simulink model "TRN_current"  (Simulink 6.2)
settings: Solver=ode45  SolverMode=SingleTasking  StartTime=0  StopTime=6  MaxStep=0.1  RelTol=1e-3  AbsTol=1e-3
libraries: simulink x1
(part 3 of 3)

== system TRN_current/Basal Ganglia/STN/STN discrete model/2 input channel1/leaky integration ==
  Inport : Inport  Port=1  LatchInput=off
  Gain : Gain  Gain=A_rate  SaturateOnIntegerOverflow=on
  Integrator : Integrator
  decay const : Gain  Orientation=left  Gain=-A_rate  SaturateOnIntegerOverflow=on
  sum : Sum  SaturateOnIntegerOverflow=on  InputSameDT=on
  Outport : Outport  InitialOutput=0
  wires:
  Gain/1 -> sum/1
  Inport/1 -> Gain/1
  Integrator/1 -> decay const/1, Outport/1
  sum/1 -> Integrator/1
  decay const/1 -> sum/2

== system TRN_current/Basal Ganglia/STN/STN discrete model/2 input channel2/input summation ==
  x1 : Inport  Port=1  LatchInput=off
  x2 : Inport  Port=2  LatchInput=off
  x3 : Inport  Port=3  LatchInput=off
  Sum : Sum  Inputs=+++  SaturateOnIntegerOverflow=on  InputSameDT=on
  W1 : Gain  Gain=W_sal  SaturateOnIntegerOverflow=on
  W2 : Gain  Gain=W_GPe  SaturateOnIntegerOverflow=on
  W3 : Gain  Gain=W_Ctx  SaturateOnIntegerOverflow=on
  out_1 : Outport  InitialOutput=0
  wires:
  Sum/1 -> out_1/1
  x1/1 -> W1/1
  x2/1 -> W2/1
  W1/1 -> Sum/1
  W2/1 -> Sum/2
  x3/1 -> W3/1
  W3/1 -> Sum/3

== system TRN_current/Basal Ganglia/STN/STN discrete model/2 input channel2/leaky integration ==
  Inport : Inport  Port=1  LatchInput=off
  Gain : Gain  Gain=A_rate  SaturateOnIntegerOverflow=on
  Integrator : Integrator
  decay const : Gain  Orientation=left  Gain=-A_rate  SaturateOnIntegerOverflow=on
  sum : Sum  SaturateOnIntegerOverflow=on  InputSameDT=on
  Outport : Outport  InitialOutput=0
  wires:
  decay const/1 -> sum/2
  sum/1 -> Integrator/1
  Integrator/1 -> Outport/1, decay const/1
  Inport/1 -> Gain/1
  Gain/1 -> sum/1

== system TRN_current/Basal Ganglia/STN/STN discrete model/2 input channel3/input summation ==
  x1 : Inport  Port=1  LatchInput=off
  x2 : Inport  Port=2  LatchInput=off
  x3 : Inport  Port=3  LatchInput=off
  Sum : Sum  Inputs=+++  SaturateOnIntegerOverflow=on  InputSameDT=on
  W1 : Gain  Gain=W_sal  SaturateOnIntegerOverflow=on
  W2 : Gain  Gain=W_GPe  SaturateOnIntegerOverflow=on
  W3 : Gain  Gain=W_Ctx  SaturateOnIntegerOverflow=on
  out_1 : Outport  InitialOutput=0
  wires:
  W3/1 -> Sum/3
  x3/1 -> W3/1
  W2/1 -> Sum/2
  W1/1 -> Sum/1
  x2/1 -> W2/1
  x1/1 -> W1/1
  Sum/1 -> out_1/1

== system TRN_current/Basal Ganglia/STN/STN discrete model/2 input channel3/leaky integration ==
  Inport : Inport  Port=1  LatchInput=off
  Gain : Gain  Gain=A_rate  SaturateOnIntegerOverflow=on
  Integrator : Integrator
  decay const : Gain  Orientation=left  Gain=-A_rate  SaturateOnIntegerOverflow=on
  sum : Sum  SaturateOnIntegerOverflow=on  InputSameDT=on
  Outport : Outport  InitialOutput=0
  wires:
  Gain/1 -> sum/1
  Inport/1 -> Gain/1
  Integrator/1 -> decay const/1, Outport/1
  sum/1 -> Integrator/1
  decay const/1 -> sum/2

== system TRN_current/Basal Ganglia/STN/STN discrete model/2 input channel4/input summation ==
  x1 : Inport  Port=1  LatchInput=off
  x2 : Inport  Port=2  LatchInput=off
  x3 : Inport  Port=3  LatchInput=off
  Sum : Sum  Inputs=+++  SaturateOnIntegerOverflow=on  InputSameDT=on
  W1 : Gain  Gain=W_sal  SaturateOnIntegerOverflow=on
  W2 : Gain  Gain=W_GPe  SaturateOnIntegerOverflow=on
  W3 : Gain  Gain=W_Ctx  SaturateOnIntegerOverflow=on
  out_1 : Outport  InitialOutput=0
  wires:
  Sum/1 -> out_1/1
  x1/1 -> W1/1
  x2/1 -> W2/1
  W1/1 -> Sum/1
  W2/1 -> Sum/2
  x3/1 -> W3/1
  W3/1 -> Sum/3

== system TRN_current/Basal Ganglia/STN/STN discrete model/2 input channel4/leaky integration ==
  Inport : Inport  Port=1  LatchInput=off
  Gain : Gain  Gain=A_rate  SaturateOnIntegerOverflow=on
  Integrator : Integrator
  decay const : Gain  Orientation=left  Gain=-A_rate  SaturateOnIntegerOverflow=on
  sum : Sum  SaturateOnIntegerOverflow=on  InputSameDT=on
  Outport : Outport  InitialOutput=0
  wires:
  decay const/1 -> sum/2
  sum/1 -> Integrator/1
  Integrator/1 -> Outport/1, decay const/1
  Inport/1 -> Gain/1
  Gain/1 -> sum/1

== system TRN_current/Basal Ganglia/STN/STN discrete model/2 input channel5/input summation ==
  x1 : Inport  Port=1  LatchInput=off
  x2 : Inport  Port=2  LatchInput=off
  x3 : Inport  Port=3  LatchInput=off
  Sum : Sum  Inputs=+++  SaturateOnIntegerOverflow=on  InputSameDT=on
  W1 : Gain  Gain=W_sal  SaturateOnIntegerOverflow=on
  W2 : Gain  Gain=W_GPe  SaturateOnIntegerOverflow=on
  W3 : Gain  Gain=W_Ctx  SaturateOnIntegerOverflow=on
  out_1 : Outport  InitialOutput=0
  wires:
  W3/1 -> Sum/3
  x3/1 -> W3/1
  W2/1 -> Sum/2
  W1/1 -> Sum/1
  x2/1 -> W2/1
  x1/1 -> W1/1
  Sum/1 -> out_1/1

== system TRN_current/Basal Ganglia/STN/STN discrete model/2 input channel5/leaky integration ==
  Inport : Inport  Port=1  LatchInput=off
  Gain : Gain  Gain=A_rate  SaturateOnIntegerOverflow=on
  Integrator : Integrator
  decay const : Gain  Orientation=left  Gain=-A_rate  SaturateOnIntegerOverflow=on
  sum : Sum  SaturateOnIntegerOverflow=on  InputSameDT=on
  Outport : Outport  InitialOutput=0
  wires:
  Gain/1 -> sum/1
  Inport/1 -> Gain/1
  Integrator/1 -> decay const/1, Outport/1
  sum/1 -> Integrator/1
  decay const/1 -> sum/2
